simulink model "etc"  (R2021a)
settings: Solver=ode45  StartTime=0.0  StopTime=10.0  RelTol=1e-3  EnableMultiTasking=on
model workspace: external: MAT-File throttleData.mat (data not in the file)
undefined symbols (not defined in the file or in its folder): Cs, digital_range, direction_range_analog, duty_range_analog, J, Kd, Ks, theta_eq, Ts, uint_range_10bit
libraries: adcUtils x2, SignalEditorBlockLib x2
settings Model: Creator=jrivitus  LastModifiedBy=sdauvill
settings SolverCC: MaxConsecutiveZCs=25  AlgebraicLoopSolver=TrustRegion
settings DataIOCC: LimitDataPoints=on  SaveFormat=Array  SaveOutput=off  SaveTime=off  ReturnWorkspaceOutputs=off
settings OptimizationCC: DefaultParameterBehavior=Inlined  ExpressionDepthLimit=2147483647  InitFltsAndDblsToZero=on  LifeSpan=1  EfficientTunableParamExpr=on
settings DebuggingCC: UnderspecifiedInitializationDetection=Classic  MergeDetectMultiDrivingBlocksExec=none  ParameterPrecisionLossMsg=none  FcnCallInpInsideContextMsg=warning  AllowSymbolicDim=off  StateNameClashWarn=warning  PregeneratedLibrarySubsystemCodeDiagnostic=none  SFUnexpectedBacktrackingDiag=warning  SFNoUnconditionalDefaultTransitionDiag=warning  SFExecutionAtInitializationDiag=none  SFMachineParentedDataDiag=warning  ArithmeticOperatorsInVariantConditions=warning
settings HardwareCC: ProdLongLongMode=on
settings ModelReferenceCC: PropagateSignalLabelsOutOfModel=off
settings SFSimCC: SimUseLocalCustomCode=off  MATLABDynamicMemAlloc=off
settings RTWCC: SystemTargetFile=ert.tlc  TemplateMakefile=ert_default_tmf  RTWUseLocalCustomCode=off
settings CodeAppCC: IgnoreCustomStorageClasses=off  StateflowObjectComments=on
settings ERTTargetCC: MultiwordLength=2048  GenerateSampleERTMain=on  InlinedParameterPlacement=NonHierarchical  ERTCustomFileTemplate=example_file_process.tlc  ConvertIfToSwitch=off  SuppressUnreachableDefaultCases=off
settings ConfigComp: CovSaveCumulativeToWorkspaceVar=on  CovExternalEMLEnable=off  CovSFcnEnable=off

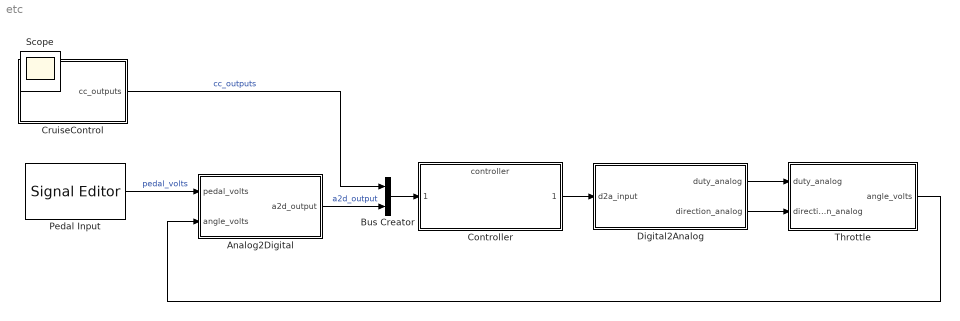
== system etc ==
  Analog2Digital : Subsystem
      settings: AttributesFormatString=(Hardware / software interface)  MinAlgLoopOccurrences=on
  Bus Creator : BusCreator  Inputs=2  OutDataTypeStr=Bus: ctrl_input_bus
  Controller : ModelReference  ModelNameDialog=controller  SimulationMode=Normal  ModelReferenceVersion=3.0
      settings: AttributesFormatString=(Software)
  CruiseControl : Subsystem
      settings: MinAlgLoopOccurrences=on
  Digital2Analog : Subsystem
      settings: AttributesFormatString=(Software / hardware interface)  MinAlgLoopOccurrences=on
  Pedal Input : SignalEditorBlockLib/Signal Editor  FileName=etc_PedalInput.mat  ActiveScenario=Group_1  ActiveSignal=Signal 1  IsBus=off  OutputBusObjectStr=Bus: BusObject  SampleTime=0  OutputAfterFinalValue=Extrapolation  Unit=inherit  PreserveSignalName=on
  Throttle : Subsystem
      settings: AttributesFormatString=(Hardware - physical system)
  Scope : Scope
  wires:
  Bus Creator/1 -> Controller/1
  Analog2Digital/1(a2d_output) -> Bus Creator/2  "a2d_output"
  CruiseControl/1(cc_outputs) -> Bus Creator/1  "cc_outputs"
  Controller/1 -> Digital2Analog/1(d2a_input)
  Digital2Analog/1(duty_analog) -> Throttle/1(duty_analog)
  Digital2Analog/2(direction_analog) -> Throttle/2(direction_analog)
  Throttle/1(angle_volts) -> Analog2Digital/2(angle_volts)
  Pedal Input/1 -> Analog2Digital/1(pedal_volts)  "pedal_volts"

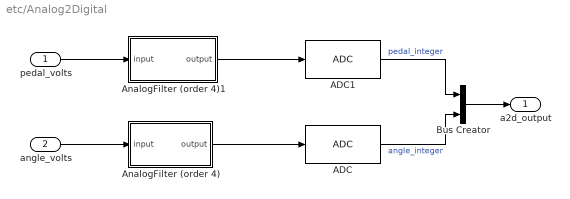
== system etc/Analog2Digital ==
  pedal_volts : Inport  OutDataTypeStr=double  PortDimensions=1  SampleTime=0
  angle_volts : Inport  Port=2  OutDataTypeStr=double  PortDimensions=1  SampleTime=0
  ADC : adcUtils/ADC  analog_range=angle_sensor_range  digital_range=uint_range_10bit  outputType=uint16  sampleRate=Ts
  ADC1 : adcUtils/ADC  analog_range=pedal_sensor_range  digital_range=uint_range_10bit  outputType=uint16  sampleRate=Ts
  AnalogFilter (order 4) : Subsystem  VariantControl=lowOrderFilter
  AnalogFilter (order 4)1 : Subsystem  VariantControl=lowOrderFilter
  Bus Creator : BusCreator  Inputs=2  OutDataTypeStr=Bus: a2d_output_bus
  a2d_output : Outport  OutDataTypeStr=Bus: a2d_output_bus  SampleTime=Ts  VectorParamsAs1DForOutWhenUnconnected=off
  wires:
  pedal_volts/1 -> AnalogFilter (order 4)1/1(input)
  angle_volts/1 -> AnalogFilter (order 4)/1(input)
  ADC1/1 -> Bus Creator/1  "pedal_integer"
  ADC/1 -> Bus Creator/2  "angle_integer"
  Bus Creator/1 -> a2d_output/1
  AnalogFilter (order 4)1/1(output) -> ADC1/1
  AnalogFilter (order 4)/1(output) -> ADC/1

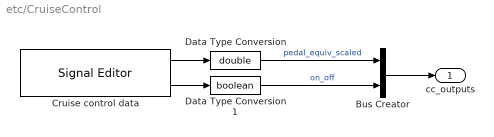
== system etc/CruiseControl ==
  Bus Creator : BusCreator  Inputs=2  OutDataTypeStr=Bus: cc_outputs_bus
  Cruise control data : SignalEditorBlockLib/Signal Editor  FileName=etc_CruiseControl_CruiseControlData.mat  ActiveScenario=Group_1  ActiveSignal=on_off  IsBus=off  OutputBusObjectStr=Bus: BusObject  SampleTime=0  OutputAfterFinalValue=Extrapolation  Unit=inherit  PreserveSignalName=on
  Data Type Conversion : DataTypeConversion  OutDataTypeStr=double  SampleTime=Ts
  Data Type Conversion1 : DataTypeConversion  OutDataTypeStr=boolean  SampleTime=Ts
  cc_outputs : Outport  OutDataTypeStr=Bus: cc_outputs_bus  SampleTime=Ts  VectorParamsAs1DForOutWhenUnconnected=off
  wires:
  Cruise control data/1 -> Data Type Conversion/1
  Cruise control data/2 -> Data Type Conversion1/1
  Data Type Conversion/1 -> Bus Creator/1  "pedal_equiv_scaled"
  Data Type Conversion1/1 -> Bus Creator/2  "on_off"
  Bus Creator/1 -> cc_outputs/1

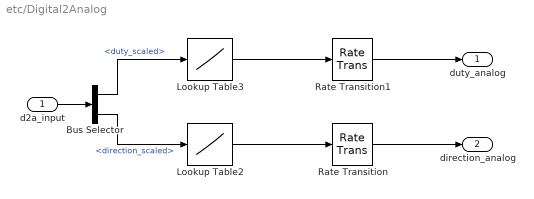
== system etc/Digital2Analog ==
  d2a_input : Inport  OutDataTypeStr=Bus: d2a_input_bus  PortDimensions=1  SampleTime=Ts
  Bus Selector : BusSelector  OutputSignals=duty_scaled,direction_scaled
  Lookup Table2 : Lookup_n-D  NumberOfTableDimensions=1  BreakpointsForDimension1=digital_range  Table=direction_range_analog  ExtrapMethod=Clip  OutDataTypeStr=double  InputSameDT=on
      settings: AttributesFormatString=Output data type: %<OutDataTypeStr>
  Lookup Table3 : Lookup_n-D  NumberOfTableDimensions=1  BreakpointsForDimension1=uint_range_10bit  Table=duty_range_analog  ExtrapMethod=Clip  OutDataTypeStr=double  InputSameDT=on
      settings: AttributesFormatString=Output data type: %<OutDataTypeStr>
  Rate Transition : RateTransition  Integrity=off  OutPortSampleTime=0
  Rate Transition1 : RateTransition  Integrity=off  OutPortSampleTime=0
  duty_analog : Outport  OutDataTypeStr=double  PortDimensions=1  SampleTime=0  VectorParamsAs1DForOutWhenUnconnected=off
  direction_analog : Outport  Port=2  OutDataTypeStr=double  PortDimensions=1  SampleTime=0  VectorParamsAs1DForOutWhenUnconnected=off
  wires:
  Bus Selector/2 -> Lookup Table2/1  "<direction_scaled>"
  Bus Selector/1 -> Lookup Table3/1  "<duty_scaled>"
  Rate Transition/1 -> direction_analog/1
  Rate Transition1/1 -> duty_analog/1
  Lookup Table3/1 -> Rate Transition1/1
  Lookup Table2/1 -> Rate Transition/1
  d2a_input/1 -> Bus Selector/1

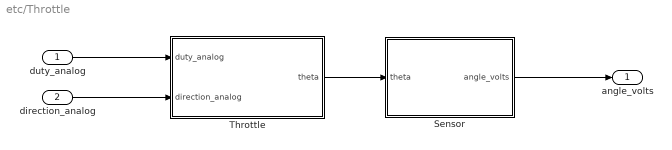
== system etc/Throttle ==
  duty_analog : Inport  OutDataTypeStr=double  PortDimensions=1  SampleTime=0
  direction_analog : Inport  Port=2  OutDataTypeStr=double  PortDimensions=1  SampleTime=0
  Sensor : Subsystem
  Throttle : Subsystem
  angle_volts : Outport  OutDataTypeStr=double  PortDimensions=1  SampleTime=0  VectorParamsAs1DForOutWhenUnconnected=off
  wires:
  duty_analog/1 -> Throttle/1(duty_analog)
  direction_analog/1 -> Throttle/2(direction_analog)
  Throttle/1(theta) -> Sensor/1(theta)
  Sensor/1(angle_volts) -> angle_volts/1

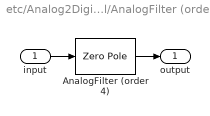
== system etc/Analog2Digital/AnalogFilter (order 4) ==
  input : Inport
  AnalogFilter (order 4) : ZeroPole  Zeros=[]  Poles=1.0e2*[-2.2739+0.6809i,-2.2739-0.6809i,-1.6518+2.0864i,-1.6518-2.0864i]  Gain=3.9899e9
  output : Outport  VectorParamsAs1DForOutWhenUnconnected=off
  wires:
  AnalogFilter (order 4)/1 -> output/1
  input/1 -> AnalogFilter (order 4)/1

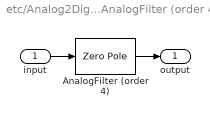
== system etc/Analog2Digital/AnalogFilter (order 4)1 ==
  input : Inport
  AnalogFilter (order 4) : ZeroPole  Zeros=[]  Poles=1.0e2*[-2.2739+0.6809i,-2.2739-0.6809i,-1.6518+2.0864i,-1.6518-2.0864i]  Gain=3.9899e9
  output : Outport  VectorParamsAs1DForOutWhenUnconnected=off
  wires:
  input/1 -> AnalogFilter (order 4)/1
  AnalogFilter (order 4)/1 -> output/1

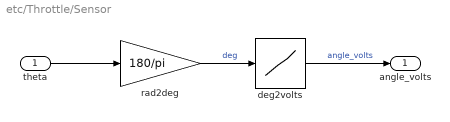
== system etc/Throttle/Sensor ==
  theta : Inport
  deg2volts : Lookup  InputValues=[0 90]  Table=[0.5 4.5]  LookUpMeth=Interpolation-Use End Values
  rad2deg : Gain  Gain=180/pi  SaturateOnIntegerOverflow=on  OutDataTypeStr=Inherit: Same as input  ParamDataTypeStr=Inherit: Same as input
  angle_volts : Outport  VectorParamsAs1DForOutWhenUnconnected=off
  wires:
  theta/1 -> rad2deg/1
  deg2volts/1 -> angle_volts/1  "angle_volts"
  rad2deg/1 -> deg2volts/1  "deg"

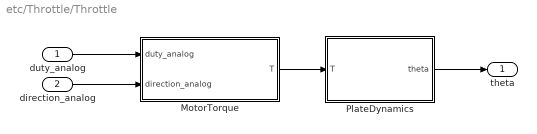
== system etc/Throttle/Throttle ==
  duty_analog : Inport
  direction_analog : Inport  Port=2
  MotorTorque : Subsystem
  PlateDynamics : Subsystem
  theta : Outport  VectorParamsAs1DForOutWhenUnconnected=off
  wires:
  MotorTorque/1(T) -> PlateDynamics/1(T)
  duty_analog/1 -> MotorTorque/1(duty_analog)
  direction_analog/1 -> MotorTorque/2(direction_analog)
  PlateDynamics/1(theta) -> theta/1

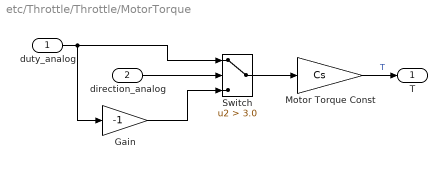
== system etc/Throttle/Throttle/MotorTorque ==
  duty_analog : Inport
  direction_analog : Inport  Port=2
  Gain : Gain  Gain=-1  SaturateOnIntegerOverflow=on  OutDataTypeStr=Inherit: Same as input  ParamDataTypeStr=Inherit: Same as input
  Motor Torque Const : Gain  Gain=Cs  SaturateOnIntegerOverflow=on  OutDataTypeStr=Inherit: Same as input  ParamDataTypeStr=Inherit: Same as input
  Switch : Switch  Criteria=u2 > Threshold  Threshold=3.0
  T : Outport  VectorParamsAs1DForOutWhenUnconnected=off
  wires:
  Switch/1 -> Motor Torque Const/1
  direction_analog/1 -> Switch/2
  duty_analog/1 -> Switch/1, Gain/1
  Gain/1 -> Switch/3
  Motor Torque Const/1 -> T/1  "T"

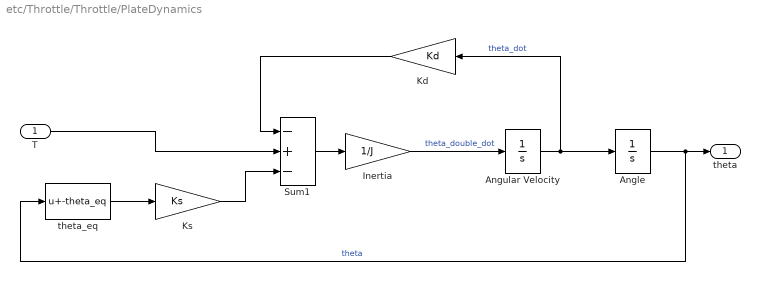
== system etc/Throttle/Throttle/PlateDynamics ==
  T : Inport
  Angle : Integrator  InitialCondition=theta_eq  LimitOutput=on  UpperSaturationLimit=pi/2  LowerSaturationLimit=0
      settings: AttributesFormatString=Initial condition: %<InitialCondition>\n%<LowerSaturationLimit> <= theta <= %<UpperSaturationLimit>
  Angular Velocity : Integrator
      settings: AttributesFormatString=Initial condition: %<InitialCondition>
  Inertia : Gain  Gain=1/J  SaturateOnIntegerOverflow=on  OutDataTypeStr=Inherit: Same as input  ParamDataTypeStr=Inherit: Same as input
  Kd : Gain  Gain=Kd  SaturateOnIntegerOverflow=on  OutDataTypeStr=Inherit: Same as input  ParamDataTypeStr=Inherit: Same as input
  Ks : Gain  Gain=Ks  SaturateOnIntegerOverflow=on  OutDataTypeStr=Inherit: Same as input  ParamDataTypeStr=Inherit: Same as input
  Sum1 : Sum  Inputs=-+-  SaturateOnIntegerOverflow=on
  theta_eq : Bias  Bias=-theta_eq
  theta : Outport  VectorParamsAs1DForOutWhenUnconnected=off
  wires:
  theta_eq/1 -> Ks/1
  Angle/1 -> theta/1, theta_eq/1  "theta"
  Angular Velocity/1 -> Angle/1, Kd/1  "theta_dot"
  Inertia/1 -> Angular Velocity/1  "theta_double_dot"
  Sum1/1 -> Inertia/1
  Kd/1 -> Sum1/1
  Ks/1 -> Sum1/3
  T/1 -> Sum1/2
